simulink model "unitstep"  (R2018b)
settings: Solver=VariableStepAuto  StartTime=0.0  StopTime=50  RelTol=1e-3
libraries: cstblocks x2
settings Model: Creator=Oguz  LastModifiedBy=Oguz

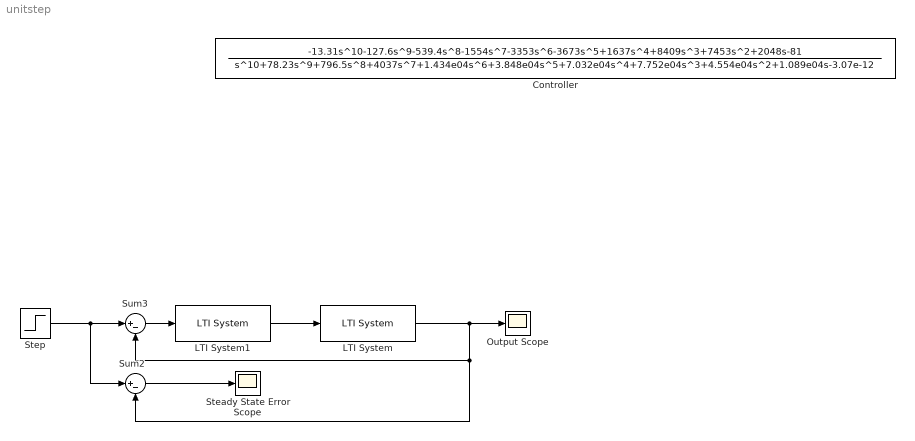
== system unitstep ==
  Controller : TransferFcn  Numerator=[-13.31 -127.6 -539.4 -1554 -3353 -3673 1637 8409 7453 2048 -81]  Denominator=[1 78.23 796.5 4037 1.434e04 3.848e04 7.032e04 7.752e04 4.554e04 1.089e04 -3.07e-12]
  LTI System : cstblocks/LTI System  sys=P  IC=[]
  LTI System1 : cstblocks/LTI System  sys=C  IC=[]
  "Output Scope " : Scope
      settings: Description=Output Scope
  Steady State Error Scope : Scope
  Step : Step  SampleTime=0
  Sum2 : Sum  Inputs=|+-
  Sum3 : Sum  Inputs=|+-
  wires:
  Sum2/1 -> Steady State Error Scope/1
  LTI System1/1 -> LTI System/1
  Step/1 -> Sum2/1, Sum3/1
  Sum3/1 -> LTI System1/1
  LTI System/1 -> "Output Scope "/1, Sum2/2, Sum3/2
